simulink model "current_coupled_thermals"  (R2025a)
settings: Solver=VariableStepAuto  StartTime=0.0  StopTime=10.0  RelTol=1e-3
libraries: myBatteries_lib x32, fl_lib x2, nesl_utility x1
settings Model: Creator=mbhattu  LastModifiedBy=mbhattu

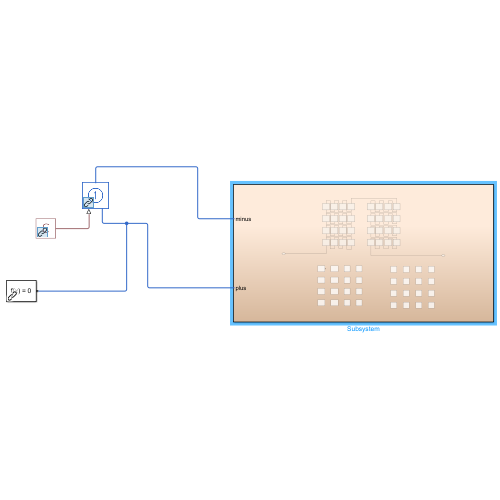
[thumbnail: Simulink's stored preview of the top-level diagram]
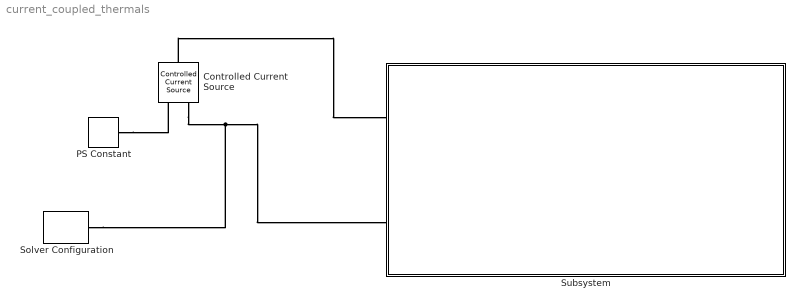
== system current_coupled_thermals ==
  Controlled Current Source : fl_lib/Electrical/Electrical Sources/Controlled Current Source
  PS Constant : fl_lib/Physical Signals/Sources/PS Constant  constant=1
  Solver Configuration : nesl_utility/Solver Configuration  PhysicalDomain=network_engine_domain  SubClassName=solver  LeftPortType=input  RightPortType=generic  Tones=[]  Harmonics=[]  SimulateNoise=off  Profile=off  UseLocalSampling=off  EnableSwitchedLinearOptims=on  FrequencyDomain=off  UseCCode=off  RelTol=0.001  AbsTol=0.001  MinStep=1e-09  ToWorkspace=off  RevertToSquareIcSolve=off  NumHomotopyIterations=100  PhasorMode=off  PhasorModeNumHarmonics=1  ConsistencySolver=NEWTON_XTOL_AFTER_FTOL  IndexReductionMethod=DerivativeReplacement  DoDC=off  ResidualTolerance=1e-09  ConsistencyTolSource=GLOBAL  ConsistencyAbsTol=0.001  ConsistencyRelTol=0.001  ConsistencyTolFactor=0.001  UseLocalSolver=off  LocalSolverChoice=NE_BACKWARD_EULER_ADVANCER  ResolveIndetEquations=on  FunctionEvalNumThread=1  LocalSolverSampleTime=0.001  DoFixedCost=off  MaxNonlinIter=3  MaxModeIter=2  ComputeImpulses=off  ImpulseIterations=2  LinearAlgebra=auto  LinearAlgebraNumThread=0  EquationFormulation=NE_TIME_EF  DelaysMemoryBudget=1024  AutomaticFiltering=on  FilteringTimeConstant=0.001  PartitionStorageMethod=AS_NEEDED  PartitionMemoryBudget=1024  PartitionMethod=ROBUST  MultibodyUseLocalSolver=off  MultibodyLocalSolverChoice=ODE1  MultibodyLocalSolverSampleTime=0.001
  Subsystem : Subsystem
  connections:
  PS Constant/RConn1 -- Controlled Current Source/RConn1
  Controlled Current Source/LConn1 -- Subsystem/LConn1
  Controlled Current Source/RConn2 -- Solver Configuration/RConn1 -- Subsystem/LConn2

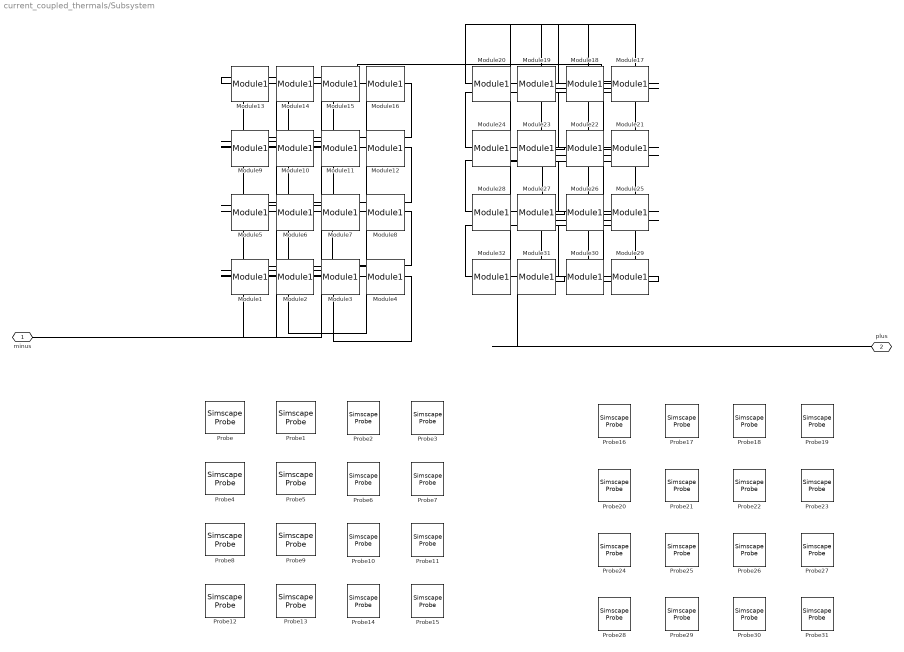
== system current_coupled_thermals/Subsystem ==
  Module{1..32} (32 alike) : myBatteries_lib/Module1  SOC_vecCell=[0, .1, .25, .5, .75, .9, 1]  V0_vecCell=[3.5057, 3.566, 3.6337, 3.7127, 3.9259, 4.0777, 4.1928] V  V_rangeCell=[0, inf] V  R0_vecCell=[.0085, .0085, .0087, .0082, .0083, .0085, .0085] Ohm  AHCell=27 A*hr  extrapolation_optionCell=simscape.enum.extrapolation.nearest  P=2  S=6  iCell_specify=off  iCell_priority=None  iCell=0 A  iCell_nominal_specify=off  iCell_nominal_value=1  iCell_nominal_unit=A  vCell_specify=off  vCell_priority=None  vCell=0 V  vCell_nominal_specify=off  vCell_nominal_value=1  vCell_nominal_unit=V  socCell_specify=off  socCell_priority=High  socCell=1  socCell_nominal_specify=off  socCell_nominal_value=1  socCell_nominal_unit=1  numCyclesCell_specify=off  numCyclesCell_priority=High  numCyclesCell=0  numCyclesCell_nominal_specify=off  numCyclesCell_nominal_value=1  numCyclesCell_nominal_unit=1  vParallelAssembly_specify=off  vParallelAssembly_priority=None  vParallelAssembly=repmat(0, 6, 1) V  vParallelAssembly_nominal_specify=off  vParallelAssembly_nominal_value=1  vParallelAssembly_nominal_unit=V  socParallelAssembly_specify=off  socParallelAssembly_priority=None  socParallelAssembly=repmat(1, 6, 1)  socParallelAssembly_nominal_specify=off  socParallelAssembly_nominal_value=1  socParallelAssembly_nominal_unit=1
      settings: InternalSimscapePortConfiguration="{\"Bottom\":[{\"id\":\"n\",\"label\":\"-\",\"type\":\"foundation.electrical.electrical\"}],\"Left\":[],\"Right\":[],\"Top\":[{\"id\":\"p\",\"label\":\"+\",\"type\":\"foundation.electrical.electrical\"}]}"
  Probe : SimscapeProbe  BoundBlock=24  Variables="{\"Cell1.soc\":{\"Probing\":\"ON\"}}"
  Probe1 : SimscapeProbe  BoundBlock=25
  Probe10 : SimscapeProbe  BoundBlock=18
  Probe11 : SimscapeProbe  BoundBlock=19
  Probe12 : SimscapeProbe  BoundBlock=12
  Probe13 : SimscapeProbe  BoundBlock=13
  Probe14 : SimscapeProbe  BoundBlock=14
  Probe15 : SimscapeProbe  BoundBlock=15
  Probe16 : SimscapeProbe  BoundBlock=47
  Probe17 : SimscapeProbe  BoundBlock=46
  Probe18 : SimscapeProbe  BoundBlock=45
  Probe19 : SimscapeProbe  BoundBlock=44
  Probe2 : SimscapeProbe  BoundBlock=26
  Probe20 : SimscapeProbe  BoundBlock=51
  Probe21 : SimscapeProbe  BoundBlock=50
  Probe22 : SimscapeProbe  BoundBlock=49
  Probe23 : SimscapeProbe  BoundBlock=48
  Probe24 : SimscapeProbe  BoundBlock=55
  Probe25 : SimscapeProbe  BoundBlock=54
  Probe26 : SimscapeProbe  BoundBlock=53
  Probe27 : SimscapeProbe  BoundBlock=52
  Probe28 : SimscapeProbe  BoundBlock=59
  Probe29 : SimscapeProbe  BoundBlock=58
  Probe3 : SimscapeProbe  BoundBlock=27
  Probe30 : SimscapeProbe  BoundBlock=57
  Probe31 : SimscapeProbe  BoundBlock=56
  Probe4 : SimscapeProbe  BoundBlock=20
  Probe5 : SimscapeProbe  BoundBlock=21
  Probe6 : SimscapeProbe  BoundBlock=22
  Probe7 : SimscapeProbe  BoundBlock=23
  Probe8 : SimscapeProbe  BoundBlock=16
  Probe9 : SimscapeProbe  BoundBlock=17
  minus : PMIOPort  Side=Left
  plus : PMIOPort  Port=2  Side=Left
  connections:
  minus/RConn1 -- Module1/RConn1
  Module1/LConn1 -- Module2/RConn1
  Module2/LConn1 -- Module3/RConn1
  Module3/LConn1 -- Module4/RConn1
  Module4/LConn1 -- Module5/RConn1
  Module5/LConn1 -- Module6/RConn1
  Module6/LConn1 -- Module7/RConn1
  Module7/LConn1 -- Module8/RConn1
  Module8/LConn1 -- Module9/RConn1
  Module9/LConn1 -- Module10/RConn1
  Module10/LConn1 -- Module11/RConn1
  Module11/LConn1 -- Module12/RConn1
  Module12/LConn1 -- Module13/RConn1
  Module13/LConn1 -- Module14/RConn1
  Module14/LConn1 -- Module15/RConn1
  Module15/LConn1 -- Module16/RConn1
  Module16/LConn1 -- Module17/RConn1
  Module17/LConn1 -- Module18/RConn1
  Module18/LConn1 -- Module19/RConn1
  Module19/LConn1 -- Module20/RConn1
  Module20/LConn1 -- Module21/RConn1
  Module21/LConn1 -- Module22/RConn1
  Module22/LConn1 -- Module23/RConn1
  Module23/LConn1 -- Module24/RConn1
  Module24/LConn1 -- Module25/RConn1
  Module25/LConn1 -- Module26/RConn1
  Module26/LConn1 -- Module27/RConn1
  Module27/LConn1 -- Module28/RConn1
  Module28/LConn1 -- Module29/RConn1
  Module29/LConn1 -- Module30/RConn1
  Module30/LConn1 -- Module31/RConn1
  Module31/LConn1 -- Module32/RConn1
  plus/RConn1 -- Module32/LConn1
